simulink model "car_speed_control_uart_proto2_2"  (R2024b)
settings: Solver=FixedStepAuto  StartTime=0.0  StopTime=500  FixedStep=0.001  RelTol=1e-3  EnableMultiTasking=on
libraries: arduinolib x2
settings Model: ExtModeTrigDuration=2  Creator=USER  LastModifiedBy=USER
settings SolverCC: AutoInsertRateTranBlk=on
settings OptimizationCC: EnhancedBackFolding=on  PassReuseOutputArgsAs=Individual arguments  ZeroExternalMemoryAtStartup=off  ZeroInternalMemoryAtStartup=off  MaxStackSize=64  OptimizeBlockOrder=speed  DifferentSizesBufferReuse=on  OptimizationCustomize=off  EfficientTunableParamExpr=on
settings DebuggingCC: ParameterTunabilityLossMsg=error
settings HardwareCC: ProdBitPerInt=16  ProdBitPerPointer=16  ProdBitPerSizeT=16  ProdBitPerPtrDiffT=16  ProdLargestAtomicFloat=None  ProdWordSize=8  ProdHWDeviceType=Atmel->AVR
settings SFSimCC: MATLABDynamicMemAlloc=off
settings RTWCC: Description=Embedded Coder  SystemTargetFile=ert.tlc  HardwareBoard=Arduino Mega 2560  TemplateMakefile=ert_default_tmf  Toolchain=Arduino AVR  BuildConfiguration=Faster Runs
settings CodeAppCC: ForceParamTrailComments=on  IgnoreCustomStorageClasses=off  OperatorAnnotations=on  SimulinkDataObjDesc=on  SFDataObjDesc=on  InsertBlockDesc=on
settings ERTTargetCC: SupportContinuousTime=on  SupportVariableSizeSignals=on  ExtModeTransport=3  ExtModeStaticAlloc=on  ExtModeAutomaticAllocSize=off  ExtModeStaticAllocSize=2048  ExtModeMexFile=ext_xcp  ExtModeIntrfLevel=Level2 - Open  InlinedParameterPlacement=Hierarchical

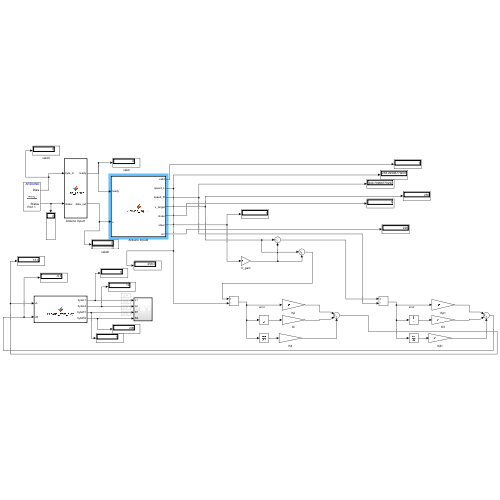
[thumbnail: Simulink's stored preview of the top-level diagram]
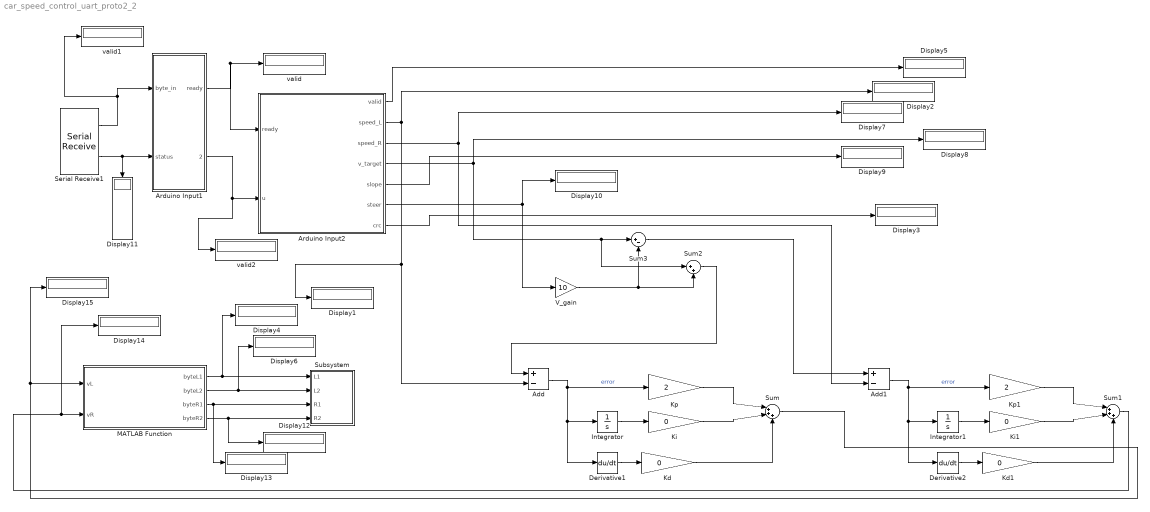
== system car_speed_control_uart_proto2_2 ==
  Add : Sum  Inputs=+-
  Add1 : Sum  Inputs=+-
  Arduino Input1 : MATLAB Function  TreatAsAtomicUnit=on
  Arduino Input2 : MATLAB Function  TreatAsAtomicUnit=on
  Derivative1 : Derivative
  Derivative2 : Derivative
  Display{1..15} (15 alike) : Display
      Display10 settings: Format=decimal (Stored Integer)
      Display2 settings: Format=decimal (Stored Integer)
      Display3 settings: Format=decimal (Stored Integer)
      Display5 settings: Format=decimal (Stored Integer)
      Display7 settings: Format=decimal (Stored Integer)
      Display8 settings: Format=decimal (Stored Integer)
      Display9 settings: Format=decimal (Stored Integer)
  Integrator : Integrator
  Integrator1 : Integrator
  Kd : Gain  Gain=0
  Kd1 : Gain  Gain=0
  Ki : Gain  Gain=0
  Ki1 : Gain  Gain=0
  Kp : Gain  Gain=2
  Kp1 : Gain  Gain=2
  MATLAB Function : MATLAB Function  TreatAsAtomicUnit=on
  Serial Receive1 : arduinolib/Serial Receive  portNumber=1  DataType=uint8  blockPlatform=ARDUINO  TimeOut=0  MaxDataLength=10  isARMArch=off  DataLengthOption=Length via dialog  Datalength=1  Header=[]  Terminator=[]  SampleTime=0.001  ShowOutStatus=on
      settings: SourceProductName=Common
  Subsystem : Subsystem  TreatAsAtomicUnit=on  SystemSampleTime=0.1
  Sum : Sum  Inputs=|+++
  Sum1 : Sum  Inputs=|+++
  Sum2 : Sum  Inputs=|++
  Sum3 : Sum  Inputs=|+-
  V_gain : Gain  Gain=10
  valid : Display
  valid1 : Display
  valid2 : Display
  wires:
  Arduino Input2/2(speed_L) -> Display2/1, Add/2, Display1/1
  Arduino Input2/4(v_target) -> Display8/1, Sum2/1, Sum3/1
  Add/1 -> Derivative1/1, Integrator/1, Kp/1  "error"
  Integrator/1 -> Ki/1
  Derivative1/1 -> Kd/1
  Kp/1 -> Sum/1
  Ki/1 -> Sum/2
  Kd/1 -> Sum/3
  Sum1/1 -> Display14/1, MATLAB Function/2(vR)
  Arduino Input1/1(ready) -> Arduino Input2/1(ready), valid/1
  Serial Receive1/2 -> Display11/1, Arduino Input1/2(status)
  Arduino Input1/2(data_out) -> valid2/1, Arduino Input2/2(u)
  Serial Receive1/1 -> valid1/1, Arduino Input1/1(byte_in)
  Arduino Input2/5(slope) -> Display9/1
  Arduino Input2/3(speed_R) -> Add1/2, Display7/1
  Arduino Input2/1(valid) -> Display5/1
  Arduino Input2/6(steer) -> Display10/1, V_gain/1
  Sum/1 -> MATLAB Function/1(vL), Display15/1
  V_gain/1 -> Sum3/2, Sum2/2
  Sum2/1 -> Add/1
  Sum3/1 -> Add1/1
  Kd1/1 -> Sum1/3
  Ki1/1 -> Sum1/2
  Kp1/1 -> Sum1/1
  Derivative2/1 -> Kd1/1
  Integrator1/1 -> Ki1/1
  Add1/1 -> Kp1/1, Integrator1/1, Derivative2/1  "error"
  MATLAB Function/1(byteL1) -> Display4/1, Subsystem/1(L1)
  MATLAB Function/2(byteL2) -> Subsystem/2(L2), Display6/1
  MATLAB Function/3(byteR1) -> Subsystem/3(R1), Display13/1
  MATLAB Function/4(byteR2) -> Display12/1, Subsystem/4(R2)
  Arduino Input2/7(crc) -> Display3/1

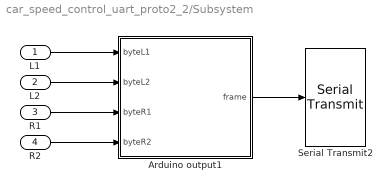
== system car_speed_control_uart_proto2_2/Subsystem ==
  L1 : Inport
  L2 : Inport  Port=2
  R1 : Inport  Port=3
  R2 : Inport  Port=4
  Arduino output1 : MATLAB Function  TreatAsAtomicUnit=on
  Serial Transmit2 : arduinolib/Serial Transmit  portNumber=1  sendmode=write  sendformat=Decimal  floatprecision=2  header=[0xAA]  terminator=[0x55]  blockPlatform=ARDUINO
      settings: SourceProductName=Common
  wires:
  L2/1 -> Arduino output1/2(byteL2)
  Arduino output1/1(frame) -> Serial Transmit2/1
  L1/1 -> Arduino output1/1(byteL1)
  R1/1 -> Arduino output1/3(byteR1)
  R2/1 -> Arduino output1/4(byteR2)

== matlab function car_speed_control_uart_proto2_2/MATLAB Function ==
  data: vL input; byteL1 output; vR input; byteL2 output; byteR1 output; byteR2 output
function [byteL1, byteL2, byteR1, byteR2] = encode_pwm_duty(vL, vR)
% 입력:
%   vL, vR: mm/s 단위의 속도값 
% 출력:
%   byteL1, byteL2: 왼쪽 듀티 (LSB, MSB)
%   byteR1, byteR2: 오른쪽 듀티 (LSB, MSB)

min_duty = 2000;
max_duty = 4000;
v_max = 400;  % 최대 속도(mm/s)

% 속도 클리핑
vL = min(max(vL, 0), v_max);
vR = min(max(vR, 0), v_max);

% 왼쪽 듀티 계산
dutyL = uint16(min_duty + (vL / v_max) * (max_duty - min_duty));
byteL2 = bitand(dutyL, 255);         % LSB
byteL1 = bitshift(dutyL, -8);        % MSB

% 오른쪽 듀티 계산
dutyR = uint16(min_duty + (vR / v_max) * (max_duty - min_duty));
byteR2 = bitand(dutyR, 255);
byteR1 = bitshift(dutyR, -8);

== matlab function car_speed_control_uart_proto2_2/Arduino Input2 ==
  data: ready input; valid output; speed_L output; speed_R output; v_target output; u input; slope output; steer output; crc output
function [valid, speed_L, speed_R, v_target, slope, steer, crc] =  Arduino_Input2( ready, u)
% UART 패킷 파서 (persistent 방식으로 이전 값 유지)
% u: [10x1] uint8, 패킷 데이터
% ready: 패킷 유효 신호

%#codegen

% 이전 출력값 저장용 persistent 변수
persistent p_valid p_speed_L p_speed_R p_v_target p_slope p_steer p_crc
 
% 초기화 (최초 실행 시)
if isempty(p_valid)
    p_valid = false;
    p_speed_L = 0.0;
    p_speed_R = 0.0;
    p_v_target = uint16(0);
    p_slope = int8(0);
    p_steer = int8(0);
    p_crc = uint8(0);
end

% 새로운 데이터가 들어왔을 경우만 업데이트
if ready == 1
    data_sum = uint16((2)) + uint16(u(3)) + uint16(u(4)) + uint16(u(5)) + uint16(u(6)) + uint16(u(7)) + uint16(u(8)) + uint16(u(9));
    if (0xFF & data_sum) == 0
        p_valid = true;
        p_speed_L = (double(u(2)) + double(u(3))/100)*10;
        p_speed_R = (double(u(4)) + double(u(5))/100)*10;
        p_v_target = (u(7))*10;
        p_slope = int8(u(6));
        p_steer = int8(u(8));
        p_crc = u(9);
    end
end

% 항상 마지막 유효 출력 반환
valid     = p_valid;
speed_L   = p_speed_L;
speed_R   = p_speed_R;
v_target  = p_v_target;
slope     = p_slope;
steer     = p_steer;
crc       = p_crc;

== matlab function car_speed_control_uart_proto2_2/Arduino Input1 ==
  data: ready output; data_out output; byte_in input; status input
function [ready, data_out] = uart_parser(byte_in, status)
% UART 프레임 수신기 (Start Byte = 0xAA, Total = 10 bytes)
% 입력: byte_in - 1바이트씩 들어오는 uint8
% 입력: status - Serial Receive의 상태 (1이면 수신 성공)
% 출력: ready - 1이면 패킷 파싱 완료
% 출력: data_out - [1x10] uint8, 패킷 데이터

persistent buffer count collecting

if isempty(buffer)
    buffer = zeros(1, 10, 'uint8');
    count = 0;
    collecting = false;
end

ready = false;
data_out = zeros(1,10,'uint8');

if status == 1
    if ~collecting
        % 아직 수집 시작 전 → start byte 찾기
        if byte_in == hex2dec('AA')
            buffer(1) = byte_in;
            count = 1;
            collecting = true;
        end
    else
    % 수집 중
    count = count + 1;
    buffer(count) = byte_in;
        if count == 10
            data_out = buffer;
            ready = true;
            count = 0;
            collecting = false;
        end
    end
end

== matlab function car_speed_control_uart_proto2_2/Subsystem/Arduino output1 ==
  data: frame output; byteL1 input; byteL2 input; byteR1 input; byteR2 input
function frame = makeFrame(byteL1, byteL2, byteR1, byteR2)
% 입력:
%   byteL1, byteL2 : 왼쪽 듀티 (LSB, MSB)
%   byteR1, byteR2 : 오른쪽 듀티 (LSB, MSB)
% 출력:
%   frame: 5-byte UART 프레임 [L_LSB, L_MSB, R_LSB, R_MSB, CRC]

% CRC 계산: 256 - mod(sum(data), 256)
data_sum = double(byteL1) + double(byteL2) + double(byteR1) + double(byteR2);
crc = mod(256 - mod(data_sum, 256), 256);

% 프레임 구성
frame = uint8([byteL1, byteL2, byteR1, byteR2, crc]);
end
